simulink model "MPC_Experiments_testing"  (R2020a)
settings: Solver=FixedStepAuto  StartTime=0.0  StopTime=tsim  FixedStep=baseRate  RelTol=1e-3  EnableMultiTasking=on
values from neighbouring files (symbols this model uses):
  Ad = dss.A    [theInitializer.m]
  ALGORITHM = 5    [Run_Initializer.m]    (also in main.m)
  baseRate = 0.05    [Run_Initializer.m]
  Bd = dss.B    [theInitializer.m]
  Cmat = zeros(6*N,9*N)    [theInitializer.m]
  con0 = [n*N, 2*N, N, N, N, N]    [Run_Initializer.m]    (also in main.m)
  drop_states_BLACK = rand([3,1])/10+init_states_BLACK    [Run_Initializer.m]
  drop_states_BLUE = rand([3,1])/10+init_states_BLUE    [Run_Initializer.m]
  drop_states_RED = rand([3,1])/10+init_states_RED    [Run_Initializer.m]
  F_thrusters_BLACK = 0.25.*ones(8,1)    [Run_Initializer.m]
  F_thrusters_BLUE = 0.25.*ones(8,1)    [Run_Initializer.m]
  F_thrusters_RED = 0.25.*ones(8,1)    [Run_Initializer.m]
  gamma = 0.95    [theInitializer.m]
  H = blkdiag(pattern{:})    [theInitializer.m]
  home_states_BLACK = [ xLength/2; yLength/2; 0]    [Run_Initializer.m]
  home_states_BLUE = [ xLength/2-0.9; yLength/2+0.5; 0]    [Run_Initializer.m]
  home_states_RED = [ xLength/2+0.7; yLength/2; pi]    [Run_Initializer.m]
  init_states_BLACK = [ct;thetat0]    [Run_Initializer.m]
  init_states_BLUE = [pobj1;0]    [Run_Initializer.m]
  init_states_RED = xi(1:3)    [Run_Initializer.m]
  Kd_tb = 0.4    [Run_Initializer.m]
  Kd_tblue = 0.4    [Run_Initializer.m]
  Kd_tr = 0.4    [Run_Initializer.m]
  Kd_xb = 5    [Run_Initializer.m]
  Kd_xblue = 5    [Run_Initializer.m]
  Kd_xr = 5    [Run_Initializer.m]
  Kd_yb = 5    [Run_Initializer.m]
  Kd_yblue = 5    [Run_Initializer.m]
  Kd_yr = 5    [Run_Initializer.m]
  KOZ_actual = KOZ + rc*sqrt(2)    [theInitializer.m]
  Kp_tb = 0.1    [Run_Initializer.m]
  Kp_tblue = 0.1    [Run_Initializer.m]
  Kp_tr = 0.1    [Run_Initializer.m]
  Kp_xb = 2    [Run_Initializer.m]
  Kp_xblue = 2    [Run_Initializer.m]
  Kp_xr = 2    [Run_Initializer.m]
  Kp_yb = 2    [Run_Initializer.m]
  Kp_yblue = 2    [Run_Initializer.m]
  Kp_yr = 2    [Run_Initializer.m]
  N = 15    [Run_Initializer.m]    (also in main.m)
  noise_variance_BLACK = 0    [Run_Initializer.m]
  noise_variance_BLUE = 0    [Run_Initializer.m]
  noise_variance_RED = 0    [Run_Initializer.m]
  Phase0_End = Phase0_Duration    (= 5)    [Run_Initializer.m]
  Phase1_End = Phase0_Duration + Phase1_Duration    (= 10)    [Run_Initializer.m]
  Phase2_End = Phase0_Duration + Phase1_Duration +                                   Phase2_Duration    (= 36)    [Run_Initializer.m]
  Phase3_End = Phase0_Duration + Phase1_Duration +                                   Phase2_Duration + Phase3_Duration    (= 166)    [Run_Initializer.m]
  Phase3_SubPhase1_End = Phase2_End + Phase3_SubPhase1_Duration    (= 40)    [Run_Initializer.m]
  Phase3_SubPhase2_End = Phase2_End + Phase3_SubPhase1_Duration +                                   Phase3_SubPhase2_Duration    (= 42)    [Run_Initializer.m]
  Phase3_SubPhase3_End = Phase2_End + Phase3_SubPhase1_Duration +                                   Phase3_SubPhase2_Duration +                                  Phase3_SubPhase3_Duration    (= 44)    [Run_Initializer.m]
  Phase3_SubPhase4_End = Phase2_End + Phase3_SubPhase1_Duration +                                   Phase3_SubPhase2_Duration +                                  Phase3_SubPhase3_Duration +                                  Phase3_SubPhase4_Duration    [Run_Initializer.m]
  Phase4_End = Phase0_Duration + Phase1_Duration +                                   Phase2_Duration + Phase3_Duration +                                   Phase4_Duration    (= 186)    [Run_Initializer.m]
  Phase5_End = Phase0_Duration + Phase1_Duration +                                   Phase2_Duration + Phase3_Duration +                                   Phase4_Duration + Phase5_Duration    (= 191)    [Run_Initializer.m]
  pobj2 = [2.0; 0.5]    [Run_Initializer.m]    (also in main.m = pobj2hz(:,2); theNonlinearConstraints0.m = pobj2hz(:,i+2))
  Q = [10,0,0,0,0,0; 0,10,0,0,0,0; 0,0,10,0,0,0; 0,0,0,300,0,0; 0,0,0,0,300,0; 0,0,0,0,0,500]    [theInitializer.m]
  R = [10,0,0; 0,10,0; 0,0,10]    [theInitializer.m]
  rcone = 0.75    [theInitializer.m]
  rdock = rt+rc+wdock    (= 0.35)    [theInitializer.m]
  serverRate = 0.1    [Run_Initializer.m]
  Sj = [KOZ_actual^(-2),0; 0,KOZ_actual^(-2)]    [theInitializer.m]
  taumax = umax*rc    (= 0.0225)    [theInitializer.m]
  Td = 2    [Run_Initializer.m]    (also in main.m)
  thetah = 20.0 * d2r    (= 0.349065850399)    [theInitializer.m]
  thetat_dot = 2.0 * d2r    (= 0.0349065850399)    [Run_Initializer.m]    (also in main.m = 2.0 * d2r)
  thruster_dist2CG_BLACK = [83.42;-52.58;55.94;-60.05;54.08;-53.92;77.06;-55.94]    [Run_Initializer.m]
  thruster_dist2CG_BLUE = [83.42;-52.58;55.94;-60.05;54.08;-53.92;77.06;-55.94]    [Run_Initializer.m]
  thruster_dist2CG_RED = [49.92;-78.08;70.46;-63.54;81.08;-50.42;57.44;-75.96]    [Run_Initializer.m]
  tol = 0.0001    [Run_Initializer.m]    (also in main.m)
  umax = 0.15    [theInitializer.m]
  vobj1 = [-0.01;0.01]    [Run_Initializer.m]    (also in main.m = [0.01;0.02])
  vobj2 = [0.0;0.0]    [Run_Initializer.m]    (also in main.m = [-0.02;-0.01])
  vtar = [0.01;0.00]    [Run_Initializer.m]    (also in main.m = [0.01;0.01])
undefined symbols (not defined in the file or in its folder): cdockoa, DiscIntNeverNeededParam, ecoa, Fmat, n, P, pdockoa, pdockr, platformSelection, simMode, Umat, WhoAmI
libraries: dspstat3 x18, raspberrypiBasiclib x10, dspsigops x9, embdlinuxlib x8, simulink x8, mspfiltlib x3, dsparch4 x3, dspswit3 x2, MainLibrary x2, sensehatlib x1
(part 10 of 10)

== matlab function MPC_Experiments_testing/Phase #3: Experiment/Change BLACK Behavior/MATLAB Function ==
  data: time input; controlx output; controlsblack parameter; controly output; controlz output
function [controlx,controly,controlz] = getControlFromDataPacket(time, controlsblack)

index = find(abs(controlsblack(:,1)-time) < 1e-5, 1);
index = index(1);

if length(index) ~= 1
    controlx = 0;
    controly = 0;
    controlz = 0;
else
    controlx = controlsblack(index,2);
    controly = controlsblack(index,3);
    controlz = controlsblack(index,4);
end

== matlab function MPC_Experiments_testing/Phase #3: Experiment/Change BLACK Behavior/Sub-Phase #4/Hough Control/MATLAB Function4 ==
  data: Oy input; e_out output; e_in input
function e_out = fcn(Oy, e_in)

a = sign(Oy'*e_in);
e_out = -a*norm(e_in);

== matlab function MPC_Experiments_testing/Phase #3: Experiment/Change BLACK Behavior/Sub-Phase #1/Hough Control/MATLAB Function2 ==
  data: Oy output; z input; Ox output
function [Oy, Ox]   = C3( z )
%C3 gives the rotation matrix about the z-axis for an angle 'z'
%   z - the angle about the z-axis which you rotate
%   A - the rotation matrix

Ox = [cos(z) sin(z); -sin(z) cos(z)]*[1;0];
Oy = [cos(z) sin(z); -sin(z) cos(z)]*[0;1];
end

== matlab function MPC_Experiments_testing/Phase #3: Experiment/Change BLACK Behavior/Sub-Phase #1/Hough Control/MATLAB Function3 ==
  data: z input; Ox output
function Ox    = C3( z )
%C3 gives the rotation matrix about the z-axis for an angle 'z'
%   z - the angle about the z-axis which you rotate
%   A - the rotation matrix

Ox = [cos(z) sin(z); -sin(z) cos(z)]*[1;0];
end

== matlab function MPC_Experiments_testing/Phase #3: Experiment/Change BLACK Behavior/Sub-Phase #1/Hough Control/MATLAB Function4 ==
  data: Oy input; e_out output; e_in input
function e_out = fcn(Oy, e_in)

a = sign(Oy'*e_in);
e_out = -a*norm(e_in);

== matlab function MPC_Experiments_testing/Phase #3: Experiment/Change BLUE Behavior/Sub-Phase #4/Hough Control/MATLAB Function3 ==
  data: z input; Ox output
function Ox    = C3( z )
%C3 gives the rotation matrix about the z-axis for an angle 'z'
%   z - the angle about the z-axis which you rotate
%   A - the rotation matrix

Ox = [cos(z) sin(z); -sin(z) cos(z)]*[1;0];
end

== matlab function MPC_Experiments_testing/Phase #3: Experiment/Change BLUE Behavior/Sub-Phase #4/Hough Control/MATLAB Function4 ==
  data: Oy input; e_out output; e_in input
function e_out = fcn(Oy, e_in)

a = sign(Oy'*e_in);
e_out = -a*norm(e_in);

== matlab function MPC_Experiments_testing/Phase #5: Hold Home/Change BLACK Behavior/Hough Control/MATLAB Function2 ==
  data: Oy output; z input; Ox output
function [Oy, Ox]   = C3( z )
%C3 gives the rotation matrix about the z-axis for an angle 'z'
%   z - the angle about the z-axis which you rotate
%   A - the rotation matrix

Ox = [cos(z) sin(z); -sin(z) cos(z)]*[1;0];
Oy = [cos(z) sin(z); -sin(z) cos(z)]*[0;1];
end

== matlab function MPC_Experiments_testing/Phase #5: Hold Home/Change BLACK Behavior/Hough Control/MATLAB Function3 ==
  data: z input; Ox output
function Ox    = C3( z )
%C3 gives the rotation matrix about the z-axis for an angle 'z'
%   z - the angle about the z-axis which you rotate
%   A - the rotation matrix

Ox = [cos(z) sin(z); -sin(z) cos(z)]*[1;0];
end

== matlab function MPC_Experiments_testing/Phase #5: Hold Home/Change BLACK Behavior/Hough Control/MATLAB Function4 ==
  data: Oy input; e_out output; e_in input
function e_out = fcn(Oy, e_in)

a = sign(Oy'*e_in);
e_out = -a*norm(e_in);

== matlab function MPC_Experiments_testing/Phase #4: Return Home/Change BLUE Behavior/Hough Control/MATLAB Function2 ==
  data: Oy output; z input; Ox output
function [Oy, Ox]   = C3( z )
%C3 gives the rotation matrix about the z-axis for an angle 'z'
%   z - the angle about the z-axis which you rotate
%   A - the rotation matrix

Ox = [cos(z) sin(z); -sin(z) cos(z)]*[1;0];
Oy = [cos(z) sin(z); -sin(z) cos(z)]*[0;1];
end

== matlab function MPC_Experiments_testing/Phase #4: Return Home/Change BLUE Behavior/Hough Control/MATLAB Function3 ==
  data: z input; Ox output
function Ox    = C3( z )
%C3 gives the rotation matrix about the z-axis for an angle 'z'
%   z - the angle about the z-axis which you rotate
%   A - the rotation matrix

Ox = [cos(z) sin(z); -sin(z) cos(z)]*[1;0];
end

== matlab function MPC_Experiments_testing/Phase #4: Return Home/Change BLUE Behavior/Hough Control/MATLAB Function4 ==
  data: Oy input; e_out output; e_in input
function e_out = fcn(Oy, e_in)

a = sign(Oy'*e_in);
e_out = -a*norm(e_in);

== matlab function MPC_Experiments_testing/Phase #5: Hold Home/Change RED Behavior/Hough Control/MATLAB Function2 ==
  data: Oy output; z input; Ox output
function [Oy, Ox]   = C3( z )
%C3 gives the rotation matrix about the z-axis for an angle 'z'
%   z - the angle about the z-axis which you rotate
%   A - the rotation matrix

Ox = [cos(z) sin(z); -sin(z) cos(z)]*[1;0];
Oy = [cos(z) sin(z); -sin(z) cos(z)]*[0;1];
end

== matlab function MPC_Experiments_testing/Phase #5: Hold Home/Change RED Behavior/Hough Control/MATLAB Function3 ==
  data: z input; Ox output
function Ox    = C3( z )
%C3 gives the rotation matrix about the z-axis for an angle 'z'
%   z - the angle about the z-axis which you rotate
%   A - the rotation matrix

Ox = [cos(z) sin(z); -sin(z) cos(z)]*[1;0];
end

== matlab function MPC_Experiments_testing/Phase #5: Hold Home/Change RED Behavior/Hough Control/MATLAB Function4 ==
  data: Oy input; e_out output; e_in input
function e_out = fcn(Oy, e_in)

a = sign(Oy'*e_in);
e_out = -a*norm(e_in);

== matlab function MPC_Experiments_testing/Phase #5: Hold Home/Change BLUE Behavior/Hough Control/MATLAB Function2 ==
  data: Oy output; z input; Ox output
function [Oy, Ox]   = C3( z )
%C3 gives the rotation matrix about the z-axis for an angle 'z'
%   z - the angle about the z-axis which you rotate
%   A - the rotation matrix

Ox = [cos(z) sin(z); -sin(z) cos(z)]*[1;0];
Oy = [cos(z) sin(z); -sin(z) cos(z)]*[0;1];
end

== matlab function MPC_Experiments_testing/Simulate Plant Dynamics/BLUE  Dynamics Model/MATLAB Function ==
  data: control_inputs input; x_ddot output; model_param parameter
function x_ddot = BLUE_dynamics(control_inputs, model_param)

%#codegen
% Fully define the size of x_ddot() for code generation:
x_ddot     = zeros(3,1);

% Extract the servicer model parameters from the model_param vector defined
% in initialize.m:
m_BLUE    = model_param(5);
I_BLUE    = model_param(6);

% Extract the control inputs from the control_input vector:
Fx        = control_inputs(1);              % [N]
Fy        = control_inputs(2);              % [N]
Tz        = control_inputs(3);              % [N.m]

% Calculate the state acceleration vector:
x_ddot(1) = Fx/m_BLUE;                      % [m/s^2]
x_ddot(2) = Fy/m_BLUE;                      % [m/s^2]
x_ddot(3) = Tz/I_BLUE;                      % [rad/s^2]

end

== matlab function MPC_Experiments_testing/Phase #5: Hold Home/Change BLUE Behavior/Hough Control/MATLAB Function3 ==
  data: z input; Ox output
function Ox    = C3( z )
%C3 gives the rotation matrix about the z-axis for an angle 'z'
%   z - the angle about the z-axis which you rotate
%   A - the rotation matrix

Ox = [cos(z) sin(z); -sin(z) cos(z)]*[1;0];
end

== matlab function MPC_Experiments_testing/Phase #5: Hold Home/Change BLUE Behavior/Hough Control/MATLAB Function4 ==
  data: Oy input; e_out output; e_in input
function e_out = fcn(Oy, e_in)

a = sign(Oy'*e_in);
e_out = -a*norm(e_in);

== matlab function MPC_Experiments_testing/From Torque, Command RW/Change RED Behavior/Calculate Saturated RPM Signal/Calculate RW RPM Increment ==
  data: Tz_Sat input; dRPM_RW output
function dRPM_RW = Calc_RW_RPM(Tz_Sat)

dRPM_RW =  (Tz_Sat/0.007244720)*(60/2/pi)*0.1;

end

== matlab function MPC_Experiments_testing/From Torque, Command RW/Change RED Behavior/Wheel RPM to PWM/Check if RW is Ready ==
  data: Status input; EnableSig output; WheelRPM_In input; WheelRPM_Out output
function [EnableSig, WheelRPM_Out] = Check_Wheel_Status(Status, WheelRPM_In)

if Status == 0
    EnableSig    = 1;
    WheelRPM_Out = WheelRPM_In;
else
    EnableSig    = 0;
    WheelRPM_Out = 0;
end

end

== matlab function MPC_Experiments_testing/From Torque, Command RW/Change RED Behavior/Wheel RPM to PWM/Get RW Direction ==
  data: MotorRPM_Sat input; WheelDirection output
function WheelDirection = GetDirection(MotorRPM_Sat)

if MotorRPM_Sat > 0
    WheelDirection = 0;
else
    WheelDirection = 1;
end
        
end

== matlab function MPC_Experiments_testing/From Torque, Command RW/Change RED Behavior/Wheel RPM to PWM/RPM to PWM Value ==
  data: MotorRPM_Sat input; MotorPWM output
function MotorPWM = RPM2PWM(MotorRPM_Sat)

PWMRange = 0.9-0.1;

MotorPWM = ((MotorRPM_Sat*PWMRange)/7000) + 0.1;

end

== matlab function MPC_Experiments_testing/Triggered Subsystem/MPC ==
  data: CONTROL output; xi input; Td parameter; N parameter; pobj2 parameter; vobj2 parameter; pdockr parameter; rdock parameter; thetah parameter; KOZ_actual parameter; Sj parameter; rcone parameter; Ad parameter; con0 parameter; Cmat parameter; Umat parameter; Fmat parameter; H parameter; gamma parameter; Bd parameter; tol parameter; x0 output; rhold output; x0 input; rhold input; ALGORITHM parameter; P parameter; Q parameter; R parameter; umax parameter; taumax parameter; n parameter; ct input; pobj1 input; vtar input; vobj1 input; thetat0 input; thetat_dot input; pdockoa parameter; ecoa parameter; cdockoa parameter
function [CONTROL, x0, rhold] = MPC(xi,Td, N, pobj2, vobj2, pdockr, rdock, thetah, KOZ_actual, Sj, rcone, Ad, con0, Cmat, Umat, Fmat, H, gamma, Bd, tol, x0, rhold, ALGORITHM, P, Q, R, umax, taumax, n, ct, pobj1, vtar, vobj1, thetat0, thetat_dot, pdockoa, ecoa, cdockoa)
    % COPY-PASTED FROM LOOP IN MAIN
    d2r = pi/180;
    
    % The moving target and obstacle positions for the current sampling instant, k
    [pobj1hz, pobj2hz, ptar] = theMovingObstacleHorizonParameters(Td,N,ct,pobj1,pobj2,vtar,vobj1,vobj2);
    
    % The rotating target parameters for the current sampling instant, k
    [thetat,m1,m2,nc1,nc2,pdock,xt,cdock] = theRotatingTargetHorizonParameters(Td,N,ptar,vtar,pdockr,rhold,rdock,cdockoa,pdockoa,ecoa,thetat_dot,thetah,thetat0);
    
    % Reshape the xt variable for use in theObjectiveFunction, ignore the
    % current state and reform into [03 xt(2) 03 xt(2) 03 ... 03 xt(N+1)]
    xt9 = zeros(9,N);
    xt9(4:9,:) = xt(:,2:N+1);
    xt9 = reshape(xt9, [9*N,1]);
    
%     if ALGORITHM >= 2
        % The reference trajectory of the chaser over the horizon of instant k
        pxref = theReferenceTrajectory(x0,N); % 2xN

        % The points ro on the KOZ boundaries of the obstacles over the horizon
        ro_1 = theObstacleLinearizer(pxref,pobj1hz(:,2:N+1),KOZ_actual);
        ro_2 = theObstacleLinearizer(pxref,pobj2hz(:,2:N+1),KOZ_actual);
        ro_t = theObstacleLinearizer(pxref,ptar(:,2:N+1),rhold);
%     end
    
%     if ALGORITHM >= 3
        % Reshape pdock for use in the linearized matrix constraints
        pdock9 = zeros(9,N);
        pdock9(4:5,:) = pdock(:,2:N+1);
        pdock9 = reshape(pdock9, [9*N,1]);
        
        % Make the ro_X and robj9 vectors for obstacle constraints
        ro_1_9 = zeros(9,N);
        ro_1_9(4:5,:) = ro_1;
        ro_1_9 = reshape(ro_1_9,9*N,1);

        ro_2_9 = zeros(9,N);
        ro_2_9(4:5,:) = ro_2;
        ro_2_9 = reshape(ro_2_9,9*N,1);

        ro_t_9 = zeros(9,N);
        ro_t_9(4:5,:) = ro_t;
        ro_t_9 = reshape(ro_t_9,9*N,1);

        robj1_9 = zeros(9,N);
        robj1_9(4:5,:) = pobj1hz(:,2:N+1);
        robj1_9 = reshape(robj1_9,9*N,1);

        robj2_9 = zeros(9,N);
        robj2_9(4:5,:) = pobj2hz(:,2:N+1);
        robj2_9 = reshape(robj2_9,9*N,1);

        rtar_9 = zeros(9,N);
        rtar_9(4:5,:) = ptar(:,2:N+1);
        rtar_9 = reshape(rtar_9,9*N,1);

        % Make the matrix for obstacle constraints
        S1 = Sj;
        S2 = Sj;
        St = [1/(rhold*rhold), 0; 0, 1/(rhold*rhold)];

        E1 = (ro_1 - pobj1hz(:,2:N+1)).' * S1;
        E2 = (ro_2 - pobj2hz(:,2:N+1)).' * S2;
        Et = (ro_t - ptar(:,2:N+1)).' * St;

        D1 = zeros(N,(9*N));
        D2 = zeros(N,(9*N));
        Dt = zeros(N,(9*N));
        for row = 1:N
            D1(row,4+(row-1)*9:5+(row-1)*9) = E1(row,:);
            D2(row,4+(row-1)*9:5+(row-1)*9) = E2(row,:);
            Dt(row,4+(row-1)*9:5+(row-1)*9) = Et(row,:);
        end   
%     end
    
    % Define the b vector for Cx = b dynamics constraint
    bvec = zeros(6*N,1);
    bvec(1:6) = Ad*xi;
    
    % Define arrays for the hyperplane normal arrays to be used for the entry cone constraints
%     if ALGORITHM == 0 || ALGORITHM == 1 || ALGORITHM == 2
%         nc1m = zeros(N,2*N);
%         nc2m = zeros(N,2*N);  
%     elseif ALGORITHM >= 3
        nc1m = zeros(N,9*N);
        nc2m = zeros(N,9*N);
%     end
        
    % Determine if the entry cone constraints should be on
    if (xi(1:2) - cdock(1:2,1)).' * (xi(1:2) - cdock(1:2,1)) < rcone*rcone % if chaser is within rcone range
        withEntryCone = 1; % turn on
        con = [n*N, 2*N, N, N, N, N, N, N];
        
%         if ALGORITHM == 0 || ALGORITHM == 1 || ALGORITHM == 2
%             % Create Nx2N matrix of the entry cone normal to each hyperplane
%             % Should be in the form
%             % ncm = [nx1 ny1  0   0   0   0  ... 0   0   0
%             %         0   0  nx2 ny2  0   0  ... 0   0   0
%             %                           ...
%             %         0   0   0   0   0   0  ... 0  nxN nyN ]
%             for i=1:N
%                 nc1m(i,2*i-1) = nc1(i+1,1);
%                 nc1m(i,2*i) = nc1(i+1,2);
% 
%                 nc2m(i,2*i-1) = nc2(i+1,1);
%                 nc2m(i,2*i) = nc2(i+1,2);
%             end
%         elseif ALGORITHM >= 3
            % Create Nx2N matrix of the entry cone normal to each hyperplane
            % Should be in the form
            % ncm = [ 0_1x3 n1_1x2 0_1x4 0_1x3  0_1x2 0_1x4  ... 0_1x3 0_1x2 0_1x4
            %         0_1x3  0_1x2 0_1x4 0_1x3 n2_1x2 0_1x4  ... 0_1x3 0_1x2 0_1x4
            %                           ...
            %         0_1x3  0_1x2 0_1x4 0_1x3  0_1x2 0_1x4  ... 0_1x3 nN+1_1x2 0_1x4
            for i=1:N
                nc1m(i,4+(i-1)*9:5+(i-1)*9) = nc1(i+1,:);
                nc2m(i,4+(i-1)*9:5+(i-1)*9) = nc2(i+1,:);
            end
%         end
        
        
    else
        withEntryCone = 0; % turn off
        con = con0;
        
        % FOR PLOTTING PURPOSES
        m1 = NaN;
        m2 = NaN;
    end
    
%     if ALGORITHM == 3
%         % Constraint Matrix
%         if ~withEntryCone
%             Wmat = [Cmat;Umat;-2*D1;-2*D2;-2*Dt];
%         else
%             Wmat = [Cmat;Umat;-2*D1;-2*D2;-2*Dt;-nc1m;nc2m];
%         end
%     elseif ALGORITHM == 4 || ALGORITHM == 5     
        % Constraint Matrix
        if ~withEntryCone
            Wmat = [-2*D1;-2*D2;-2*Dt];
        else
            Wmat = [-2*D1;-2*D2;-2*Dt;-nc1m;nc2m];
        end
%     end
    
    % Objective Function
%     if ALGORITHM == 0
%         ofun = @(x) theObjectiveFunction0(x,N,xt,P,Q,R);
%     elseif ALGORITHM > 0
%         ofun = @(x)theObjectiveFunction123(x,xt9,H);
%     end
    
    % Nonlinear Constraints (cl <= nlcon(x) <= cu)
%     if ALGORITHM == 0
%         nlcon = @(x) theNonlinearConstraints0(x,N,Ad,Bd,xi,Sj,...
%             pobj1hz,pobj2hz,ct,nc1,nc2,pdock,withEntryCone,rhold);
%     elseif ALGORITHM == 1
%         nlcon = @(x) theNonlinearConstraints1(x,N,Ad,Cmat,xi,...
%             pobj1hz,pobj2hz,ct,nc1m,nc2m,pdock,withEntryCone,KOZ_actual,rhold);
%     elseif ALGORITHM == 2
%         nlcon = @(x) theNonlinearConstraints2(x,N,bvec,...
%             Cmat,con0,pobj1hz,pobj2hz,nc1m,nc2m,pdock,withEntryCone,ro_1,ro_2,...
%             ro_t,ptar,KOZ_actual,rhold);
%     elseif ALGORITHM == 3
%         nlcon = @(x) theNonlinearConstraints3(x,Wmat);
%     end
    
    % Constraint upper and lower limits
%     if ALGORITHM == 0 || ALGORITHM == 1 || ALGORITHM == 2  
%         [cl,cu] = theConstraintLimits012(con0,con,umax,taumax);
%     elseif ALGORITHM == 3   
%         [cl,cu] = theConstraintLimits3(con0,con,bvec,Fmat,D1,D2,Dt,...
%             ro_1_9,ro_2_9,ro_t_9,robj1_9,robj2_9,rtar_9,nc1m,nc2m,pdock9);
%     elseif ALGORITHM == 4 || ALGORITHM == 5
        [cl,cu,bineqvec] = theConstraintLimits4(Umat,Fmat,Wmat,con0,con,...
            D1,D2,Dt,ro_1_9,ro_2_9,ro_t_9,robj1_9,robj2_9,rtar_9,nc1m,...
            nc2m,pdock9);
%     end
    
    % Setup Options
%     if ALGORITHM < 4
%         opts = 0;
% %         opts = optiset('solver','ipopt','display','final','maxiter',50);
%     elseif ALGORITHM == 4
%         options = optimoptions('fmincon','Algorithm','sqp','MaxIterations',50);
%     elseif ALGORITHM == 5
        options = optimoptions('quadprog','Algorithm','active-set','MaxIterations',50);
%     end

%     if ALGORITHM < 4    
%         % Computing the gradient and jacobian -- Complex Step Differentiation
%         grad = @(x) cstepJac(ofun,x);
%         jac = @(x) cstepJac(nlcon,x);
%         % Build OPTI Problem
%         Opt = opti('fun',ofun,'grad',grad,'nl',nlcon,cl,cu,'jac',jac,'x0',x0,'options',opts);
%     end
    
    % Solve!
%     if ALGORITHM < 4
        %tic
%         [x,fval,ef,info] = solve(Opt,x0);
        %solCPUtime(end+1) = toc;
        0;
%     elseif ALGORITHM == 4
        %tic
%         x = fmincon(ofun,x0,Wmat,bineqvec,Cmat,bvec,cl,cu,[],options);
        %solCPUtime(end+1) = toc;
%     elseif ALGORITHM == 5
        %tic
        [x,fval] = quadprog(H,-H.'*xt9,Wmat,bineqvec,Cmat,bvec,cl,cu,x0,options);
        %solCPUtime(end+1) = toc;
%     end
   

    % Save data
%     sol(end+1:end+9) = x(1:9);
%     soliter(1:n,count) = xi;
%     soliter(n+1:n+9*N,count) = x;
%     solpobj(count,1) = pobj1hz(1,1); 
%     solpobj(count,2) = pobj1hz(2,1);
%     solpobj(count,3) = pobj2hz(1,1);
%     solpobj(count,4) = pobj2hz(2,1);
%     solptar(count,1) = ptar(1,1);
%     solptar(count,2) = ptar(2,1);
%     solm1(count,1) = m1(1);
%     solm2(count,1) = m2(1);
%     solthetat(count,1) = thetat(1);
%     solpdock(count,1:2) = pdock(:,1);
%     if ALGORITHM == 0
%         solJ(end+1) = theObjectiveFunction0(x,N,xt,P,Q,R);
%     elseif ALGORITHM > 0
%         solJ(end+1) = theObjectiveFunction123(x,xt9,H);
%     end
%     count = count + 1;

    CONTROL = x(1:3);
    
    % Determine if the chaser is docked using the 'current' positions of
    % the chaser and docking condition; done using only position
    if (xi(1:2) - cdock(1:2,1)).' * (xi(1:2) - cdock(1:2,1)) < tol
        isdocked = 1;
    end
    
    % Set the next guess as the solution from the previous iteration
    xi = x(4:9); % the next 'current' state of the chaser spacecraft
    x0 = [x(10:end);0;0;0;Ad*x0(4+9*(N-2):9+9*(N-2)) + Bd*x0(1+9*(N-1):3+9*(N-1))];
    %x0(1:9) = [];
    %x0(end+1:end+3) = [0,0,0].';
    
    % THIS IS NEW (16 FEB 2022, NOT IN ARCHIVED FILES)
    %x0(end+1:end+n) = Ad*x0(4+9*(N-2):9+9*(N-2)) + Bd*x0(1+9*(N-1):3+9*(N-1));
    
    % Update rhold if:
    %  - the position of the chaser matches the holding position, within tolerance
    %  - the attitude of the chaser matches the docking condition, within tolerance
    %  - the holding radius is larger than its minimum allowable size, rdock
    if abs((xi(1:2) - xt(1:2,1)).' * (xi(1:2) - xt(1:2,1))) < 0.5 % if position error is below tolerance
        if abs(xi(3) - cdock(3,1)) < 10*d2r % if attitude error is below tolerance
            if rhold > rdock
                rhold = rhold * gamma; % decrease the holding radius
                if rhold < rdock
                    rhold = rdock; % set to the minimum holding radius, rdock
                end
            end
        end
    end
    
    % Set the next 'current' target and obstacle positions
%     ct = ptar(:,2);
%     pobj1 = pobj1hz(:,2); 
%     pobj2 = pobj2hz(:,2);
        
    % Set the new target theta value for the next iteration
%     thetat0 = thetat(2);
    
end

== matlab function MPC_Experiments_testing/Simulate Plant Dynamics/RED Dynamics Model/MATLAB Function ==
  data: control_inputs input; x_ddot output; model_param parameter
function x_ddot = RED_dynamics(control_inputs, model_param)

%#codegen
% Fully define the size of x_ddot() for code generation:
x_ddot     = zeros(3,1);

% Extract the servicer model parameters from the model_param vector defined
% in initialize.m:
m_RED    = model_param(1);
I_RED    = model_param(2);

% Extract the control inputs from the control_input vector:
Fx        = control_inputs(1);              % [N]
Fy        = control_inputs(2);              % [N]
Tz        = control_inputs(3);              % [N.m]

% Calculate the state acceleration vector:
x_ddot(1) = Fx/m_RED;                      % [m/s^2]
x_ddot(2) = Fy/m_RED;                      % [m/s^2]
x_ddot(3) = Tz/I_RED;                      % [rad/s^2]

end

== matlab function MPC_Experiments_testing/Gyroscope & Acceleration Algorithms/Change RED Behavior/Create Rotation Matrix ==
  data: Rz input; C_Ib output
function C_Ib = RotateFrame(Rz)

C_bI = [  cos(Rz) sin(Rz)
         -sin(Rz) cos(Rz) ];

C_Ib = inv(C_bI);

end

== matlab function MPC_Experiments_testing/Gyroscope & Acceleration Algorithms/Change BLACK Behavior/Create Rotation Matrix ==
  data: Rz input; C_Ib output
function C_Ib = RotateFrame(Rz)

C_bI = [  cos(Rz) sin(Rz)
         -sin(Rz) cos(Rz) ];

C_Ib = inv(C_bI);

end

== matlab function MPC_Experiments_testing/Gyroscope & Acceleration Algorithms/Change RED Behavior/ChangeOrientation ==
  data: u input; y output
function y = ChangeOrientation(u)

y = rotz(-90)*u';

== matlab function MPC_Experiments_testing/Gyroscope & Acceleration Algorithms/Change BLACK Behavior/ChangeOrientation ==
  data: u input; y output
function y = ChangeOrientation(u)

y = rotz(-90)*u';

== matlab function MPC_Experiments_testing/Gyroscope & Acceleration Algorithms/Change BLUE Behavior/ChangeOrientation ==
  data: u input; y output
function y = ChangeOrientation(u)

y = rotz(-90)*u';

== matlab function MPC_Experiments_testing/Gyroscope & Acceleration Algorithms/Change BLUE Behavior/Create Rotation Matrix ==
  data: Rz input; C_Ib output
function C_Ib = RotateFrame(Rz)

C_bI = [  cos(Rz) sin(Rz)
         -sin(Rz) cos(Rz) ];

C_Ib = inv(C_bI);

end

== matlab function MPC_Experiments_testing/Phase #3: Experiment/Change BLACK Behavior/Sub-Phase #3 /Hough Control/MATLAB Function2 ==
  data: Oy output; z input; Ox output
function [Oy, Ox]   = C3( z )
%C3 gives the rotation matrix about the z-axis for an angle 'z'
%   z - the angle about the z-axis which you rotate
%   A - the rotation matrix

Ox = [cos(z) sin(z); -sin(z) cos(z)]*[1;0];
Oy = [cos(z) sin(z); -sin(z) cos(z)]*[0;1];
end

== matlab function MPC_Experiments_testing/Phase #3: Experiment/Change BLACK Behavior/Sub-Phase #3 /Hough Control/MATLAB Function3 ==
  data: z input; Ox output
function Ox    = C3( z )
%C3 gives the rotation matrix about the z-axis for an angle 'z'
%   z - the angle about the z-axis which you rotate
%   A - the rotation matrix

Ox = [cos(z) sin(z); -sin(z) cos(z)]*[1;0];
end

== matlab function MPC_Experiments_testing/Phase #3: Experiment/Change BLACK Behavior/Sub-Phase #3 /Hough Control/MATLAB Function4 ==
  data: Oy input; e_out output; e_in input
function e_out = fcn(Oy, e_in)

a = sign(Oy'*e_in);
e_out = -a*norm(e_in);

== matlab function MPC_Experiments_testing/Simulate Plant Dynamics/BLACK Dynamics Model/MATLAB Function ==
  data: control_inputs input; x_ddot output; model_param parameter
function x_ddot = BLACK_dynamics(control_inputs, model_param)

%#codegen
% Fully define the size of x_ddot() for code generation:
x_ddot     = zeros(3,1);

% Extract the servicer model parameters from the model_param vector defined
% in initialize.m:
m_BLACK    = model_param(3);
I_BLACK    = model_param(4);

% Extract the control inputs from the control_input vector:
Fx        = control_inputs(1);              % [N]
Fy        = control_inputs(2);              % [N]
Tz        = control_inputs(3);              % [N.m]

% Calculate the state acceleration vector:
x_ddot(1) = Fx/m_BLACK;                      % [m/s^2]
x_ddot(2) = Fy/m_BLACK;                      % [m/s^2]
x_ddot(3) = Tz/I_BLACK;                      % [rad/s^2]

end

== matlab function MPC_Experiments_testing/Phase #3: Experiment/Change BLACK Behavior/Sub-Phase #2 /Hough Control/MATLAB Function2 ==
  data: Oy output; z input; Ox output
function [Oy, Ox]   = C3( z )
%C3 gives the rotation matrix about the z-axis for an angle 'z'
%   z - the angle about the z-axis which you rotate
%   A - the rotation matrix

Ox = [cos(z) sin(z); -sin(z) cos(z)]*[1;0];
Oy = [cos(z) sin(z); -sin(z) cos(z)]*[0;1];
end

== matlab function MPC_Experiments_testing/Phase #3: Experiment/Change BLACK Behavior/Sub-Phase #2 /Hough Control/MATLAB Function3 ==
  data: z input; Ox output
function Ox    = C3( z )
%C3 gives the rotation matrix about the z-axis for an angle 'z'
%   z - the angle about the z-axis which you rotate
%   A - the rotation matrix

Ox = [cos(z) sin(z); -sin(z) cos(z)]*[1;0];
end

== matlab function MPC_Experiments_testing/Phase #3: Experiment/Change BLACK Behavior/Sub-Phase #2 /Hough Control/MATLAB Function4 ==
  data: Oy input; e_out output; e_in input
function e_out = fcn(Oy, e_in)

a = sign(Oy'*e_in);
e_out = -a*norm(e_in);

== matlab function MPC_Experiments_testing/Simulate Plant Dynamics/Sample and Hold Data to Match PhaseSpace (BLUE)/MATLAB Function ==
  data: TIME input; y output; SERVER input
function y = fcn(TIME, SERVER)

if mod(TIME,SERVER) == 0
    y = 1;
else
    y = 0;
end

== matlab function MPC_Experiments_testing/From Force//Torque to PWM Signal/Change BLUE Behavior/Calculate Thruster ON//OFF/MATLAB Function ==
  data: H output; thruster_dist2CG_BLUE parameter; F_thrusters_BLUE parameter
function H = MakeH(thruster_dist2CG_BLUE,F_thrusters_BLUE)

Vec1 = [ -1
         -1
          0 
          0
          1
          1
          0
          0 ];
      
Vec2 = [  0
          0
          1
          1
          0
          0
         -1
         -1 ];
     
Vec3 = thruster_dist2CG_BLUE./1000;

Mat1 = [Vec1, Vec2, Vec3]';

Mat2 = diag((F_thrusters_BLUE./2));

H    = Mat1*Mat2;

end

== matlab function MPC_Experiments_testing/From Force//Torque to PWM Signal/Change BLUE Behavior/Calculate Thruster ON//OFF/MATLAB Function1 ==
  data: H output; thruster_dist2CG_BLUE parameter; F_thrusters_BLUE parameter
function H = MakeH(thruster_dist2CG_BLUE,F_thrusters_BLUE)

Vec1 = [ -1
         -1
          0 
          0
          1
          1
          0
          0 ];
      
Vec2 = [  0
          0
          1
          1
          0
          0
         -1
         -1 ];
     
Vec3 = thruster_dist2CG_BLUE./1000;

Mat1 = [Vec1, Vec2, Vec3]';

Mat2 = diag((F_thrusters_BLUE./2));

H    = Mat1*Mat2;

end
